simulink model "simulateASK"  (R2017a)
settings: Solver=VariableStepAuto  StartTime=0.0  StopTime=inf  RelTol=1e-3
InitFcn:
  | fs = 1e5;
  | Ts = 1/fs;
  | Tb = 0.001;
  | frameSize = 100;
libraries: commfilt2 x3, dsparch4 x2, commsink2 x2, dspsrcs4 x2, commchan3 x1, commrandsrc3 x1
settings Model: SimulationMode=accelerator  Creator=prust  LastModifiedBy=prust

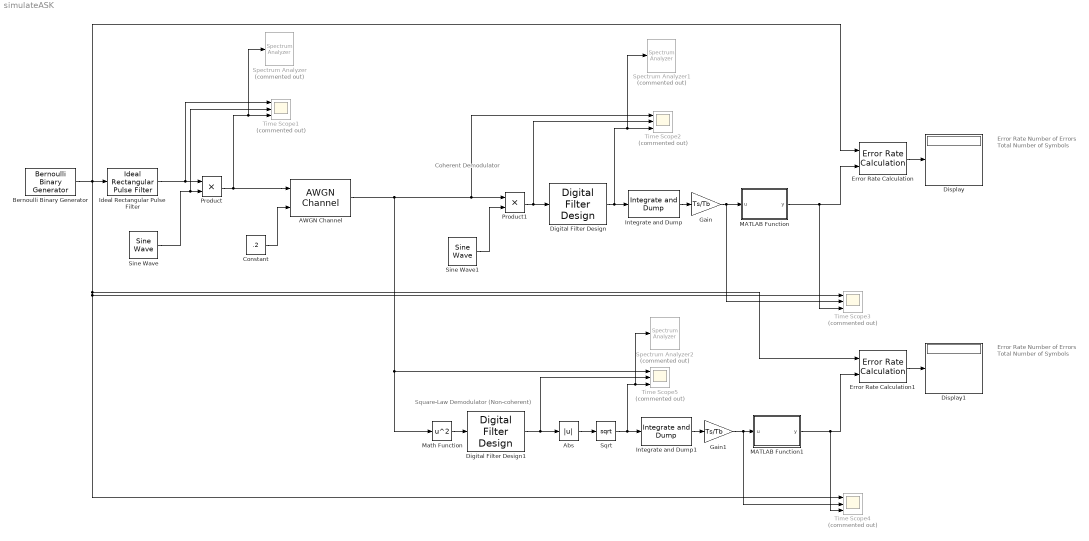
== system simulateASK ==
  note: Square-Law Demodulator (Non-coherent)
  note: Coherent Demodulator
  note: Error Rate
      |
      | Number of Errors
      |
      | Total Number of Symbols
  note: Error Rate
      |
      | Number of Errors
      |
      | Total Number of Symbols
  AWGN Channel : commchan3/AWGN Channel  InputProcessing=Columns as channels (frame based)  seed=67  noiseMode=Variance from port  EbNodB=12  EsNodB=10  SNRdB=10  bitsPerSym=1  Ps=1  Tsym=1/1000  variance=1
  Abs : Abs
  Bernoulli Binary Generator : commrandsrc3/Bernoulli Binary Generator  ProbabilityOfZero=0.5  SeedSource=Auto  Seed=0  SampleTime=Tb  SamplesPerFrame=frameSize  OutputDataType=double  SimulateUsing=Interpreted execution
  Constant : Constant  Value=.2
  Digital Filter Design : dsparch4/Digital Filter Design  mwdsp_browser_bugfix_var=off
  Digital Filter Design1 : dsparch4/Digital Filter Design  mwdsp_browser_bugfix_var=off
  Display : Display
  Display1 : Display
  Error Rate Calculation : commsink2/Error Rate Calculation  N=1  st_delay=0  cp_mode=Entire frame  subframe=[]  PMode=Port  WsName=ErrorVec  RsMode2=off  stop=off  numErr=100  maxBits=1e6
  Error Rate Calculation1 : commsink2/Error Rate Calculation  N=1  st_delay=0  cp_mode=Entire frame  subframe=[]  PMode=Port  WsName=ErrorVec  RsMode2=off  stop=off  numErr=100  maxBits=1e6
  Gain : Gain  Gain=Ts/Tb
  Gain1 : Gain  Gain=Ts/Tb
  Ideal Rectangular Pulse Filter : commfilt2/Ideal Rectangular Pulse Filter  pulseLen=Tb/Ts  pulseDelay=0  InputProcessing=Columns as channels (frame based)  RateOptions=Enforce single-rate processing  sampMode=Mute  normCheck=off  normMode=Sum of samples  filterGain=1  saveAsFlag=0  roundingMode=Floor  overflowMode=off  firstCoeffDataTypeStr=Inherit: Same word length as input  firstCoeffMin=[]  firstCoeffMax=[]  firstCoeffLastDataTypeStr=Inherit: Same word length as input  outputDataTypeStr=Inherit: Same as accumulator  outputMin=[]  outputMax=[]  outputLastDataTypeStr=Inherit: Same as accumulator
      settings: SourceProductName=Communications System Toolbox  SourceProductBaseCode=CM
  Integrate and Dump : commfilt2/Integrate and Dump  obssamples=Tb/Ts  offsetsamples=50  nodump=off  roundingMode=Floor  overflowMode=off  outputDataTypeStr=Inherit: Same as accumulator  outputLastDataTypeStr=Inherit: Same as accumulator
      settings: SourceProductName=Communications System Toolbox
  Integrate and Dump1 : commfilt2/Integrate and Dump  obssamples=Tb/Ts  offsetsamples=50  nodump=off  roundingMode=Floor  overflowMode=off  outputDataTypeStr=Inherit: Same as accumulator  outputLastDataTypeStr=Inherit: Same as accumulator
      settings: SourceProductName=Communications System Toolbox
  MATLAB Function : MATLAB Function  TreatAsAtomicUnit=on
  MATLAB Function1 : MATLAB Function  TreatAsAtomicUnit=on
  Math Function : Math  Operator=square  SaturateOnIntegerOverflow=on
  Product : Product
  Product1 : Product
  Sine Wave : dspsrcs4/Sine Wave  Amplitude=sqrt(2)  Frequency=10e3  Phase=0  SampleMode=Discrete  OutComplex=Real  CompMethod=Trigonometric fcn  TableSize=Speed  SampleTime=1/fs  SamplesPerFrame=frameSize*Tb/Ts  ResetState=Restart at time zero  OutputFrames=off  dataType=double  wordLen=16  udDataType=sfix(16)  fracBitsMode=Best precision  numFracBits=15  OutDataTypeStr=double  LastOutDataTypeStr=double
  Sine Wave1 : dspsrcs4/Sine Wave  Amplitude=sqrt(2)  Frequency=10e3  Phase=0  SampleMode=Discrete  OutComplex=Real  CompMethod=Trigonometric fcn  TableSize=Speed  SampleTime=1/fs  SamplesPerFrame=frameSize*Tb/Ts  ResetState=Restart at time zero  OutputFrames=off  dataType=double  wordLen=16  udDataType=sfix(16)  fracBitsMode=Best precision  numFracBits=15  OutDataTypeStr=double  LastOutDataTypeStr=double
  Spectrum Analyzer : SpectrumAnalyzer  Commented=on
  Spectrum Analyzer1 : SpectrumAnalyzer  Commented=on
  Spectrum Analyzer2 : SpectrumAnalyzer  Commented=on
  Sqrt : Sqrt  SaturateOnIntegerOverflow=on
  Time Scope{1..5} (5 alike) : Scope  Commented=on  NumInputPorts=3
  wires:
  Bernoulli Binary Generator/1 -> Time Scope3/1, Time Scope4/1, Error Rate Calculation1/1, Error Rate Calculation/1, Ideal Rectangular Pulse Filter/1
  Ideal Rectangular Pulse Filter/1 -> Time Scope1/1, Product/1
  Sine Wave/1 -> Time Scope1/2, Product/2
  Product/1 -> Spectrum Analyzer/1, Time Scope1/3, AWGN Channel/1
  AWGN Channel/1 -> Math Function/1, Time Scope5/1, Time Scope2/1, Product1/1
  Sine Wave1/1 -> Product1/2
  Product1/1 -> Time Scope2/2, Digital Filter Design/1
  Digital Filter Design/1 -> Spectrum Analyzer1/1, Time Scope2/3, Integrate and Dump/1
  Error Rate Calculation/1 -> Display/1
  Integrate and Dump/1 -> Gain/1
  Gain/1 -> MATLAB Function/1(u), Time Scope3/2
  MATLAB Function/1(y) -> Time Scope3/3, Error Rate Calculation/2
  Constant/1 -> AWGN Channel/2
  Math Function/1 -> Digital Filter Design1/1
  Digital Filter Design1/1 -> Time Scope5/2, Abs/1
  Abs/1 -> Sqrt/1
  Sqrt/1 -> Spectrum Analyzer2/1, Time Scope5/3, Integrate and Dump1/1
  Integrate and Dump1/1 -> Gain1/1
  Gain1/1 -> Time Scope4/2, MATLAB Function1/1(u)
  MATLAB Function1/1(y) -> Error Rate Calculation1/2, Time Scope4/3
  Error Rate Calculation1/1 -> Display1/1

== matlab function simulateASK/MATLAB Function1 ==
  data: u input; y output
function y = fcn(u)
u(u<0.5) = 0;
u(u>=0.5) = 1;
y = u;

== matlab function simulateASK/MATLAB Function ==
  data: u input; y output
function y = fcn(u)
u(u<0.5) = 0;
u(u>=0.5) = 1;
y = u;
